simulink model "kinematic_model"  (R2020b)
settings: Solver=ode4  StartTime=0.0  StopTime=9.10  FixedStep=0.001  RelTol=1e-3
undefined symbols (not defined in the file or in its folder): THETA_ref, X_ref, Y_ref
settings Model: Creator=salvatore  LastModifiedBy=salvatore

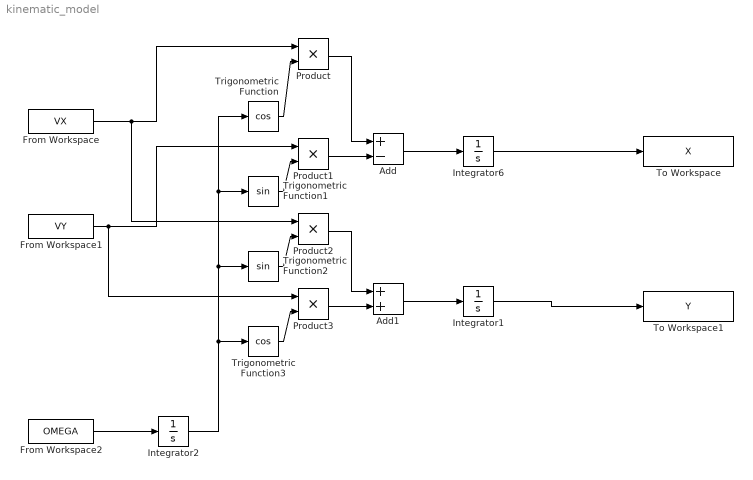
== system kinematic_model ==
  Add : Sum  Inputs=+-
  Add1 : Sum
  From Workspace : FromWorkspace  VariableName=VX
  From Workspace1 : FromWorkspace  VariableName=VY
  From Workspace2 : FromWorkspace  VariableName=OMEGA
  Integrator1 : Integrator  InitialCondition=Y_ref(1)
  Integrator2 : Integrator  InitialCondition=THETA_ref(1)
  Integrator6 : Integrator  InitialCondition=X_ref(1)
  Product{,1..3} (4 alike) : Product
  To Workspace : ToWorkspace  VariableName=X  SampleTime=-1
  To Workspace1 : ToWorkspace  VariableName=Y  SampleTime=-1
  Trigonometric Function : Trigonometry  Operator=cos
  Trigonometric Function1 : Trigonometry
  Trigonometric Function2 : Trigonometry
  Trigonometric Function3 : Trigonometry  Operator=cos
  wires:
  Integrator2/1 -> Trigonometric Function/1, Trigonometric Function1/1, Trigonometric Function2/1, Trigonometric Function3/1
  Trigonometric Function/1 -> Product/2
  Trigonometric Function1/1 -> Product1/2
  Trigonometric Function2/1 -> Product2/2
  Trigonometric Function3/1 -> Product3/2
  From Workspace/1 -> Product2/1, Product/1
  From Workspace1/1 -> Product3/1, Product1/1
  From Workspace2/1 -> Integrator2/1
  Integrator1/1 -> To Workspace1/1
  Integrator6/1 -> To Workspace/1
  Product/1 -> Add/1
  Product1/1 -> Add/2
  Product2/1 -> Add1/1
  Product3/1 -> Add1/2
  Add1/1 -> Integrator1/1
  Add/1 -> Integrator6/1
